simulink model "pade2"  (Simulink 8.1)
settings: Solver=ode4  StartTime=0.0  StopTime=10.0  FixedStep=0.001  RelTol=1e-3
values from neighbouring files (symbols this model uses):
  a = 0.378726441955    [pade2.mat]    (also in pade2_errc.m = x0(1))
  b = 1.03008381562    [pade2.mat]    (also in pade2_errc.m = x0(2))
  padel = [1 -20.6844037735 192.530051759 -929.219510127 1922.03515417]    [pade2.mat]
  padem = [1 20.6844037735 192.530051759 929.219510127 1922.03515417]    [pade2.mat]
settings Model: Creator=student  LastModifiedBy=adasdeb
settings DataIOCC: LimitDataPoints=off
settings DebuggingCC: FcnCallInpInsideContextMsg=EnableAllAsWarning
settings GRTTargetCC: CombineOutputUpdateFcns=on  GRTInterface=off

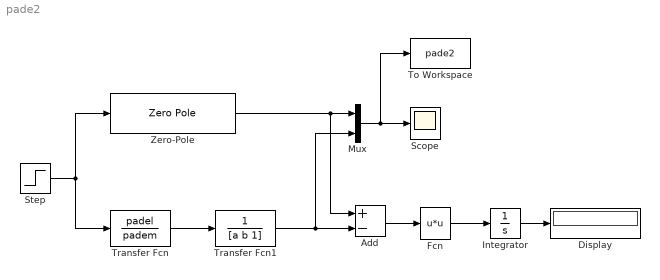
== system pade2 ==
  Add : Sum  Inputs=+-
  Display : Display
  Fcn : Fcn  Expr=u*u
  Integrator : Integrator
  Mux : Mux  Inputs=2
  Scope : Scope
  Step : Step  Time=0  SampleTime=0
  To Workspace : ToWorkspace  VariableName=pade2  SampleTime=-1
  Transfer Fcn : TransferFcn  Numerator=padel  Denominator=padem
  Transfer Fcn1 : TransferFcn  Denominator=[a b 1]
  Zero-Pole : ZeroPole  Zeros=[]  Poles=linspace(-5,-5,10)  Gain=5^10
  wires:
  Step/1 -> Transfer Fcn/1, Zero-Pole/1
  Transfer Fcn/1 -> Transfer Fcn1/1
  Zero-Pole/1 -> Mux/1, Add/1
  Transfer Fcn1/1 -> Mux/2, Add/2
  Integrator/1 -> Display/1
  Mux/1 -> To Workspace/1, Scope/1
  Add/1 -> Fcn/1
  Fcn/1 -> Integrator/1
